simulink model "systemHeat"  (R2017a)
settings: Solver=VariableStepAuto  StartTime=0.0  StopTime=1000000  FixedStep=1  RelTol=1e-3
values from neighbouring files (symbols this model uses):
  A = [-(h+k/delta)*cons1 k/delta*cons1 0 0 ... (first row only)    [listVariables.m]
  B = [1 0 0; 0 0 0; 0 0 0; 0 1 1]    [listVariables.m]
settings Model: Creator=PC  LastModifiedBy=Student

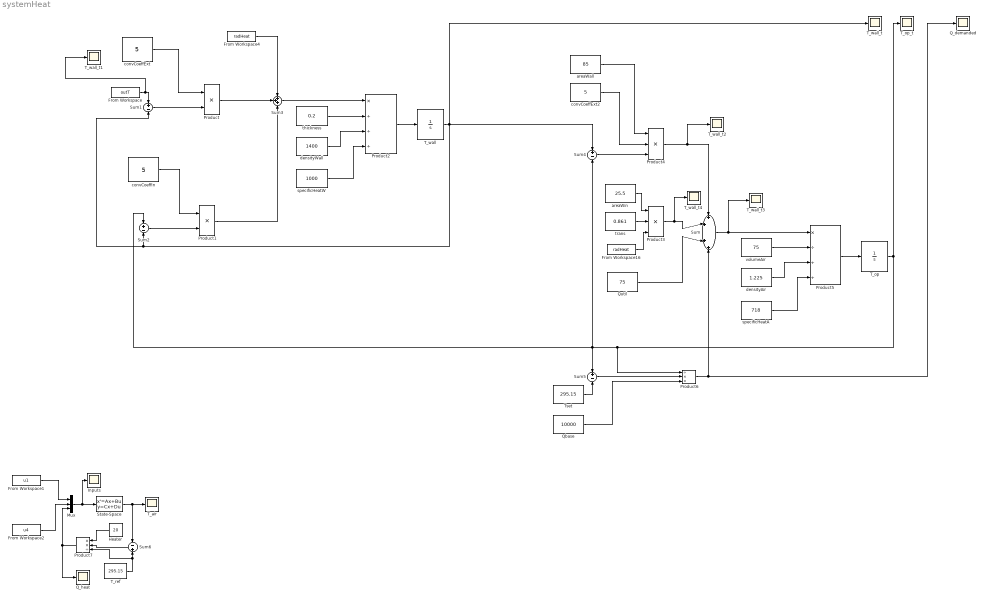
== system systemHeat ==
  From Workspace : FromWorkspace  VariableName=outT  SampleTime=0
  From Workspace1 : FromWorkspace  VariableName=u1  SampleTime=0
  From Workspace16 : FromWorkspace  VariableName=radHeat  SampleTime=0
  From Workspace2 : FromWorkspace  VariableName=u4  SampleTime=0
  From Workspace4 : FromWorkspace  VariableName=radHeat  SampleTime=0
  Heater : Constant  Value=20
  Inputs : Scope
  Mux : Mux  Inputs=3
  Product : Product
  Product1 : Product
  Product2 : Product  Inputs=*///
  Product3 : Product  Inputs=3
  Product4 : Product  Inputs=3
  Product5 : Product  Inputs=*///
  Product6 : Product  Inputs=/**
  Product7 : Product  Inputs=**/
  Q_demanded : Scope
  Q_heat : Scope
  Qbase : Constant  Value=10000
  Qutil : Constant  Value=75
  State-Space : StateSpace  A=A  B=B  C=[0 0 0 1]  D=[0 0 0]  X0=[270; 275; 280; 285]
  Sum : Sum  Inputs=++++
  Sum{1..2,4..5} (4 alike) : Sum  Inputs=+-
  Sum3 : Sum  Inputs=+++
  Sum6 : Sum  Inputs=-+
  T_air : Scope
  T_op : Integrator  InitialCondition=290.15
  T_op_t : Scope
  T_ref : Constant  Value=295.15
  T_wall : Integrator  InitialCondition=293.15
  T_wall_t{,1..4} (5 alike) : Scope
  Tset : Constant  Value=295.15
  areaWall : Constant  Value=85
  areaWin : Constant  Value=25.5
  convCoeffExt : Constant  Value=5
  "convCoeffExt2 " : Constant  Value=5
  convCoeffIn : Constant  Value=5
  densityAir : Constant  Value=1.225
  densityWall : Constant  Value=1400
  specificHeatA : Constant  Value=718
  specificHeatW : Constant  Value=1000
  thickness : Constant  Value=0.2
  trans : Constant  Value=0.861
  volumeAir : Constant  Value=75
  wires:
  From Workspace/1 -> T_wall_t1/1, Sum1/1
  Sum1/1 -> Product/2
  convCoeffExt/1 -> Product/1
  Sum2/1 -> Product1/2
  T_op/1 -> Product6/1, Sum4/2, Sum5/1, Sum2/1, T_op_t/1
  Product/1 -> Sum3/2
  Product1/1 -> Sum3/3
  thickness/1 -> Product2/2
  densityWall/1 -> Product2/3
  specificHeatW/1 -> Product2/4
  Sum3/1 -> Product2/1
  Product2/1 -> T_wall/1
  From Workspace4/1 -> Sum3/1
  T_wall/1 -> Sum4/1, T_wall_t/1, Sum1/2, Sum2/2
  Sum4/1 -> Product4/3
  "convCoeffExt2 "/1 -> Product4/2
  areaWall/1 -> Product4/1
  areaWin/1 -> Product3/1
  trans/1 -> Product3/2
  From Workspace16/1 -> Product3/3
  Product4/1 -> T_wall_t2/1, Sum/1
  Product3/1 -> T_wall_t4/1, Sum/2
  Qutil/1 -> Sum/3
  specificHeatA/1 -> Product5/4
  densityAir/1 -> Product5/3
  Product5/1 -> T_op/1
  volumeAir/1 -> Product5/2
  Sum/1 -> T_wall_t3/1, Product5/1
  Tset/1 -> Sum5/2
  Sum5/1 -> Product6/2
  Qbase/1 -> Product6/3
  Product6/1 -> Q_demanded/1, Sum/4
  convCoeffIn/1 -> Product1/1
  From Workspace1/1 -> Mux/1
  Mux/1 -> Inputs/1, State-Space/1
  State-Space/1 -> Sum6/1, T_air/1
  From Workspace2/1 -> Mux/2
  T_ref/1 -> Product7/3, Sum6/2
  Product7/1 -> Q_heat/1, Mux/3
  Sum6/1 -> Product7/2
  Heater/1 -> Product7/1
